simulink model "F16ASYM_Controlled_AoA"  (R2012b)
settings: Solver=ode3  SolverMode=SingleTasking  StartTime=0.0  StopTime=inf  FixedStep=T_sim  RelTol=1e-3
InitFcn:
  | load('NN_c_weights_Last_stable.mat')
values from neighbouring files (symbols this model uses):
  K_b_AoA = params(3)    [Cost_function.m]
  K_b_q = params(4)    [Cost_function.m]
  learning = 20    [Scheduling_desing.m]
  Model_used_flag = 1    [Scheduling_desing.m]
  reg_param = 0.5    [Scheduling_desing.m]
  T_sim = 0.02    [Scheduling_desing.m]
  tau_AoA = params(1)    [Cost_function.m]
  tau_q = params(2)    [Cost_function.m]
  Theta_1_roll_last = [0.00183613313267 0.00115998993235 0.0006676025148 0.00194921904952 0.00134963559861 0.00034352059664 0.000447169388141 0.00146749660935 0.00110199952389 7.77922383894e-05 0.00109492833348 0.00192687590535 ... (360 elements, 30x12)]    [NN_i_weights_LAST_STABLE.mat]
  Theta_2_roll_last = [0.000469743069697 0.000355923851088 0.00180035760697 0.00191855117771 0.00118851504447 0.0013331642065 0.0013164316578 0.000643981263341 0.00176817665434 0.000113802099363 0.000426534542462 0.00113815782354 ... (620 elements, 20x31)]    [NN_i_weights_LAST_STABLE.mat]
  Theta_3_roll_last = [9.62071520568e-05 -0.000389870886846 2.08260845013e-05 0.000140787743673 -0.000917525755397 -0.0014324207578 -0.00154701573815 -0.00131544476264 -0.00101205584381 5.06515794689e-05 -0.00111443483676 -0.00143957416141 ... (21 elements, 1x21)]    [NN_i_weights_LAST_STABLE.mat]
  V_long_lastA_w_z = [0.352826086601 -0.253633004548 -0.642535042878 0.237749930435 -0.618390629538 0.858074761295 0.268211230628 -0.448715080196 -0.0406384631192 0.401147605577 0.60598427709 0.0500551915851 ... (300 elements, 30x10)]    [NN_i_weights_LAST_STABLE.mat]
  V_long_lastAoA = [0.0774300162379 0.0911421319631 0.0352371192557 0.0542170286952 0.0651171200844 0.0177112012707 0.0982957728448 0.000259994642558 0.0194724569123 0.0466321328252 0.0556687953852 0.0252668067142 ... (300 elements, 30x10)]    [NN_i_weights_LAST_STABLE.mat]
  V_roll_last = [0.0540918675943 0.0557493347212 0.0839792276608 0.0460576391794 0.0671229058124 0.100220403067 0.0722493281881 0.0648875457457 0.00447599349201 0.0607299103823 0.0488037966361 0.0176785979393 ... (360 elements, 30x12)]    [NN_i_weights_LAST_STABLE.mat]
  V_yaw_last = [0.0965149149679 0.00833616709545 0.0365734360076 0.0523944217566 0.00790252078455 0.0700053845887 0.0345164868709 0.0111568465295 0.094060639546 0.0205483560006 0.000798047494256 0.0862769385758 ... (360 elements, 30x12)]    [NN_i_weights_LAST_STABLE.mat]
  velocity = M_eval_sche(I,J)*a    [Scheduling_desing.m]
  W_long_lastA_w_z = [-0.0522913429974 0.00385484301394 -0.00465489482472 -0.0139416219936 0.00295196421483 -0.013027768541 0.00585545058915 0.00278802233571 -0.00906272782329 -0.000396112031465 0.00405849743321 0.00509668457818 ... (31 elements, 1x31)]    [NN_i_weights_LAST_STABLE.mat]
  W_long_lastAoA = [-0.0192589013922 0.00873109909713 0.00432649597332 0.0420946902441 0.0293366820194 0.0351497798191 0.0234952374236 0.0360841187718 0.0112233388211 0.030147202199 0.0369533138617 0.00218839076415 ... (31 elements, 1x31)]    [NN_i_weights_LAST_STABLE.mat]
  W_roll_last = [-0.0006515532842 0.000535485585715 0.000550946920743 0.000806030945453 0.00045976209382 0.00065557954304 0.000945902185602 0.00070191398535 0.000635215543728 4.66501377412e-05 0.000597079583757 0.000485790566765 ... (31 elements, 1x31)]    [NN_i_weights_LAST_STABLE.mat]
  W_yaw_last = [-4.34263633305e-05 8.83823048922e-05 1.65575463724e-05 3.60293102233e-05 5.19752447623e-05 7.06399280852e-06 7.02425975821e-05 3.62680255076e-05 1.29996379937e-05 8.05072914397e-05 2.39941870661e-05 2.52427840574e-06 ... (31 elements, 1x31)]    [NN_i_weights_LAST_STABLE.mat]
undefined symbols (not defined in the file or in its folder): a1, alpha_map_eval, B, beta_map_eval, C_L_0, DiscIntNeverNeededParam, fi_flag_Simulink, G_eval, H_sq, H_sq_autotrim, k_B, m_B, M_sq, M_sq_autotrim, sigbuilder_block, Stall_curve, trim_control, trim_state, trim_throttle, V_Comp_A_w_z_last, V_Comp_last, V_roll_lastMOD, W_Comp_A_w_z_last, W_Comp_last, W_roll_lastMOD
libraries: Adaptive_FaultTolerantControl x43, dspsigops x29, F16_Actuator_Library x14, simulink x8, aerolibatmos2 x7, dsparch4 x6, simulink_extras x5, aerolibtransform2 x5, qcatlib x4, dspmtrx3 x3, dspvision x2, dspsnks4 x2
(part 4 of 11)

== system F16ASYM_Controlled_AoA/Primary Controller/P controller + adaptive Crossed NN + AWU+Lim  ==
  A_w_z des : Inport
  AoA des (rad) : Inport  Port=2
  p des (rad/s) : Inport  Port=3
  beta des (rad) : Inport  Port=4
  Anti-windup A_w_z : Inport  Port=5
  Anti-windup AoA : Inport  Port=6
  Anti-windup beta : Inport  Port=7
  All measures : Inport  Port=8
  Anti-windup signals : Inport  Port=9
  Body Rates Controller : Subsystem
  Bus Creator : BusCreator  Inputs=3
  Bus Creator1 : BusCreator  Inputs=3
  Bus Creator2 : BusCreator
  Bus Creator3 : BusCreator  Inputs=2
  Bus Selector3 : BusSelector  OutputSignals=signal1.SS meas (rad)
  Complete crossed On-line (adaptive) multi-layer NN : Subsystem  Variant=on  OverrideUsingVariant=NN on AoA
      mask Display:
      | image(imread('ANN.png'))
      | 
      | port_label('input', 1, 'v prev')
      | port_label('input', 2, 'All meas')
      | port_label('input', 3, 'NN vars')
      | port_label('input', 4, 'Anti-windup')
      | 
      | port_label('output', 1, 'v_ad^')
  Constant : Constant  Value=NaN
  Display{,1..3,5..6} (6 alike) : Display
  "Display4 " : Display
  Lat_dir Dyn Inversion: beta_dot->r_c : Subsystem
  Long Dyn Inversion: alpha_dot ->q : Subsystem
  Longitudinal Controller: AoA or A_w_z : Subsystem  Variant=on  OverrideUsingVariant=Controller of AoA
  Memory : Memory  X0=[0,0,0]
  Physical limitation : Subsystem
  Ref Model and P Controller : Adaptive_FaultTolerantControl/Ref Model and P Controller  tau=0.45  y_i=trim_state(9)  K_f=1  K_b=5
  Scope1 : Scope
      settings: YMin=-8000  YMax=9000  SaveName=ScopeData27
  "Sigmoid " : Subsystem  mask{a=0.15}
      mask prompts: a "Sigmoid a param"
      mask TypeOptions a: a/Value
      mask Display:
      | x=-25:0.1:25;
      | 
      | y=(2.0 ./ (1.0 + exp(-a.*x))-1) ;
      | y2=zeros(size(x));
      | 
      | plot(x,y,x,y2);
      | 
      | text(-12,0.5, ['a= ',num2str(a)])
  Sum : Sum  Inputs=-+|
  Sum1 : Sum  Inputs=+-|
  Terminator1 : Terminator
  Angular acc des : Outport
  Control_in : Outport  Port=2
  wires:
  Lat_dir Dyn Inversion: beta_dot->r_c/1(r_c) -> Display6/1, Body Rates Controller/3(r_ref)
  Bus Selector3/1 -> Ref Model and P Controller/2  "<SS meas (rad)>"
  p des (rad/s)/1 -> Body Rates Controller/1(p_ref)
  Long Dyn Inversion: alpha_dot ->q/1(q_c) -> Body Rates Controller/2(q_ref), Display1/1
  beta des (rad)/1 -> Ref Model and P Controller/1
  Longitudinal Controller: AoA or A_w_z/3(alpha_dot_c) -> Long Dyn Inversion: alpha_dot ->q/1(alpha_dot_c), Display/1
  AoA des (rad)/1 -> Longitudinal Controller: AoA or A_w_z/2(AoA des (rad))
  Anti-windup AoA/1 -> Longitudinal Controller: AoA or A_w_z/4(Anti-windup AoA)
  Anti-windup A_w_z/1 -> Longitudinal Controller: AoA or A_w_z/3(Anti-windup A_w_z)
  A_w_z des/1 -> Longitudinal Controller: AoA or A_w_z/1(A_w_z des)
  Sum/1 -> "Display4 "/1, "Sigmoid "/1(In), Physical limitation/1(v comm)  "v"
  All measures/1 -> Complete crossed On-line (adaptive) multi-layer NN/2(All_meas), Physical limitation/2(all meas), Body Rates Controller/4(All_meas), Lat_dir Dyn Inversion: beta_dot->r_c/2(All_meas), Bus Selector3/1, Long Dyn Inversion: alpha_dot ->q/2(All_meas), Longitudinal Controller: AoA or A_w_z/5(All meas)
  Body Rates Controller/4(Angular acc des (rad/s^2)) -> Display3/1, Sum/2  "v_p+v_dot_ff"
  Bus Creator/1 -> Complete crossed On-line (adaptive) multi-layer NN/3(NN variables)
  Memory/1 -> Complete crossed On-line (adaptive) multi-layer NN/1(v_ad^ prev)
  Body Rates Controller/2(p_chanel vars) -> Bus Creator/2  "p_chanel_vars"
  Body Rates Controller/1(q_chanel vars) -> Bus Creator1/3  "q_chanel_vars"
  Longitudinal Controller: AoA or A_w_z/1(A_chanel vars) -> Bus Creator1/1  "A_chanel vars"
  Longitudinal Controller: AoA or A_w_z/2(alpha_chanel vars) -> Bus Creator1/2  "alpha_chanel vars"
  Bus Creator1/1 -> Bus Creator/1  "Long chanel"
  Ref Model and P Controller/2 -> Bus Creator2/1  "beta_sf_dot"
  Ref Model and P Controller/3 -> Sum1/1, Bus Creator2/2  "beta_sf"
  Sum1/1 -> Bus Creator2/3  "beta_err"
  Ref Model and P Controller/4 -> Sum1/2
  Ref Model and P Controller/5 -> Bus Creator2/4  "K_b_beta"
  Body Rates Controller/3(r_chanel vars) -> Bus Creator3/1  "r_chanel vars"
  Bus Creator2/1 -> Bus Creator3/2  "beta_chanel vars"
  Bus Creator3/1 -> Bus Creator/3  "beta_r_chanel"
  Anti-windup beta/1 -> Terminator1/1
  "Sigmoid "/1(Out) -> Memory/1
  Complete crossed On-line (adaptive) multi-layer NN/1(v_ad^) -> Scope1/1, Display2/1, Sum/1  "v_ad^"
  Ref Model and P Controller/1 -> Display5/1, Lat_dir Dyn Inversion: beta_dot->r_c/1(beta_dot_c)
  Anti-windup signals/1 -> Complete crossed On-line (adaptive) multi-layer NN/4(AWU)
  Physical limitation/1(v limted) -> Angular acc des/1
  Constant/1 -> Control_in/1

== system F16ASYM_Controlled_AoA/Primary Controller/P controller + adaptive Isolated NN ==
  A_w_z des : Inport
  AoA des (rad) : Inport  Port=2
  p des (rad/s) : Inport  Port=3
  beta des (rad) : Inport  Port=4
  Anti-windup A_w_z : Inport  Port=5
  Anti-windup AoA : Inport  Port=6
  Anti-windup beta : Inport  Port=7
  All measures : Inport  Port=8
  Anti-windup signals : Inport  Port=9
  Body Rates Controller : Subsystem
  Bus Creator : BusCreator  Inputs=3
  Bus Creator1 : BusCreator  Inputs=3
  Bus Creator2 : BusCreator
  Bus Creator3 : BusCreator  Inputs=2
  Bus Selector3 : BusSelector  OutputSignals=signal1.SS meas (rad)
  Display{,1..6} (7 alike) : Display
  Ground : Ground
  Lat_dir Dyn Inversion: beta_dot->r_c : Subsystem
  Long Dyn Inversion: alpha_dot ->q : Subsystem
  Longitudinal Controller: AoA or A_w_z : Subsystem  Variant=on  OverrideUsingVariant=Controller of A_w_z
  Memory : Memory  X0=[0,0,0]
  On-line (adaptive) multi-layer NNs : Subsystem
      mask Display:
      | image(imread('ANN.png'))
      | 
      | port_label('input', 1, 'v prev')
      | port_label('input', 2, 'All meas')
      | port_label('input', 3, 'NN vars')
      | 
      | port_label('output', 1, 'v_ad^')
  On-line (adaptive) multi-layer NNs SIMPL : Subsystem  Commented=on
      mask Display:
      | image(imread('ANN.png'))
      | 
      | port_label('input', 1, 'v prev')
      | port_label('input', 2, 'All meas')
      | port_label('input', 3, 'NN vars')
      | 
      | port_label('output', 1, 'v_ad^')
  Ref Model and P Controller : Adaptive_FaultTolerantControl/Ref Model and P Controller  tau=0.45  y_i=trim_state(9)  K_f=1  K_b=5
  "Sigmoid " : Subsystem  mask{a=0.15}
      mask prompts: a "Sigmoid a param"
      mask TypeOptions a: a/Value
      mask Display:
      | x=-25:0.1:25;
      | 
      | y=(2.0 ./ (1.0 + exp(-a.*x))-1) ;
      | y2=zeros(size(x));
      | 
      | plot(x,y,x,y2);
      | 
      | text(-12,0.5, ['a= ',num2str(a)])
  Sum : Sum  Inputs=-+|
  Sum1 : Sum  Inputs=+-|
  Terminator : Terminator
  Terminator1 : Terminator
  Angular acc des : Outport
  Control_in : Outport  Port=2
  wires:
  Lat_dir Dyn Inversion: beta_dot->r_c/1(r_c) -> Display6/1, Body Rates Controller/3(r_ref)
  Bus Selector3/1 -> Ref Model and P Controller/2  "<SS meas (rad)>"
  p des (rad/s)/1 -> Body Rates Controller/1(p_ref)
  Long Dyn Inversion: alpha_dot ->q/1(q_c) -> Display1/1, Body Rates Controller/2(q_ref)
  beta des (rad)/1 -> Ref Model and P Controller/1
  Longitudinal Controller: AoA or A_w_z/3(alpha_dot_c) -> Long Dyn Inversion: alpha_dot ->q/1(alpha_dot_c), Display/1
  AoA des (rad)/1 -> Longitudinal Controller: AoA or A_w_z/2(AoA des (rad))
  Anti-windup AoA/1 -> Longitudinal Controller: AoA or A_w_z/4(Anti-windup AoA)
  Anti-windup A_w_z/1 -> Longitudinal Controller: AoA or A_w_z/3(Anti-windup A_w_z)
  A_w_z des/1 -> Longitudinal Controller: AoA or A_w_z/1(A_w_z des)
  Sum/1 -> Display4/1, "Sigmoid "/1(In), Angular acc des/1  "v"
  Body Rates Controller/4(Angular acc des (rad/s^2)) -> Display3/1, Sum/2  "v_p+v_dot_ff"
  Bus Creator/1 -> On-line (adaptive) multi-layer NNs/3(NN variables)
  Memory/1 -> On-line (adaptive) multi-layer NNs/1(v_ad^ prev)
  Body Rates Controller/2(p_chanel vars) -> Bus Creator/2  "p_chanel_vars"
  Body Rates Controller/1(q_chanel vars) -> Bus Creator1/3  "q_chanel_vars"
  Longitudinal Controller: AoA or A_w_z/1(A_chanel vars) -> Bus Creator1/1  "A_chanel vars"
  Longitudinal Controller: AoA or A_w_z/2(alpha_chanel vars) -> Bus Creator1/2  "alpha_chanel vars"
  Bus Creator1/1 -> Bus Creator/1  "Long chanel"
  Ref Model and P Controller/2 -> Bus Creator2/1  "beta_sf_dot"
  Ref Model and P Controller/3 -> Sum1/1, Bus Creator2/2  "beta_sf"
  Sum1/1 -> Bus Creator2/3  "beta_err"
  Ref Model and P Controller/4 -> Sum1/2
  Ref Model and P Controller/5 -> Bus Creator2/4  "K_b_beta"
  Body Rates Controller/3(r_chanel vars) -> Bus Creator3/1  "r_chanel vars"
  Bus Creator2/1 -> Bus Creator3/2  "beta_chanel vars"
  Bus Creator3/1 -> Bus Creator/3  "beta_r_chanel"
  Anti-windup beta/1 -> Terminator1/1
  "Sigmoid "/1(Out) -> Memory/1
  On-line (adaptive) multi-layer NNs/1(v_ad^) -> Sum/1, Display2/1  "v_ad^"
  Ref Model and P Controller/1 -> Display5/1, Lat_dir Dyn Inversion: beta_dot->r_c/1(beta_dot_c)
  All measures/1 -> On-line (adaptive) multi-layer NNs/2(All_meas), Body Rates Controller/4(All_meas), Lat_dir Dyn Inversion: beta_dot->r_c/2(All_meas), Bus Selector3/1, Long Dyn Inversion: alpha_dot ->q/2(All_meas), Longitudinal Controller: AoA or A_w_z/5(All meas)
  Anti-windup signals/1 -> Terminator/1
  Ground/1 -> Control_in/1

== system F16ASYM_Controlled_AoA/Primary Controller/PI Primary Controller ==
  A_w_z des : Inport
  AoA des (rad) : Inport  Port=2
  p des (rad/s) : Inport  Port=3
  beta des (rad) : Inport  Port=4
  Anti-windup A_w_z : Inport  Port=5
  Anti-windup AoA : Inport  Port=6
  Anti-windup beta : Inport  Port=7
  All measures : Inport  Port=8
  Anti-windup signals : Inport  Port=9
  Body Rates Controller : Subsystem
  Bus Selector3 : BusSelector  OutputSignals=signal1.SS meas (rad)
  Display{,1..3} (4 alike) : Display
  Ground : Ground
  Lat_dir Dyn Inversion: beta_dot->r_c : Subsystem
  Long Dyn Inversion: alpha_dot ->q : Subsystem
  Longitudinal Controller: AoA or A_w_z : Subsystem  Variant=on  OverrideUsingVariant=Controller of A_w_z
  PI Controller: beta  controller : Adaptive_FaultTolerantControl/PI Controller  delta=0  K_a=0  y_i=trim_state(9)  Des_way=auto  omega_n=2  xi=1  Z1=-50  K_b=6  f_i=0.25  f_c=1
  Angular acc des : Outport
  Control_in : Outport  Port=2
  wires:
  A_w_z des/1 -> Longitudinal Controller: AoA or A_w_z/1(A_w_z des)
  Anti-windup A_w_z/1 -> Longitudinal Controller: AoA or A_w_z/3(Anti-windup A_w_z)
  Anti-windup AoA/1 -> Longitudinal Controller: AoA or A_w_z/4(Anti-windup AoA)
  AoA des (rad)/1 -> Longitudinal Controller: AoA or A_w_z/2(AoA des (rad))
  Longitudinal Controller: AoA or A_w_z/1(alpha_dot_c) -> Display/1, Long Dyn Inversion: alpha_dot ->q/1(alpha_dot_c)
  All measures/1 -> Bus Selector3/1, Lat_dir Dyn Inversion: beta_dot->r_c/2(All_meas), Body Rates Controller/4(All_meas), Longitudinal Controller: AoA or A_w_z/5(All meas), Long Dyn Inversion: alpha_dot ->q/2(All_meas)
  Anti-windup beta/1 -> PI Controller: beta  controller/3
  beta des (rad)/1 -> PI Controller: beta  controller/1
  Long Dyn Inversion: alpha_dot ->q/1(q_c) -> Body Rates Controller/2(q_ref), Display1/1
  p des (rad/s)/1 -> Body Rates Controller/1(p_ref)
  Body Rates Controller/1(Angular acc des (rad/s^2)) -> Angular acc des/1
  PI Controller: beta  controller/1 -> Lat_dir Dyn Inversion: beta_dot->r_c/1(beta_dot_c), Display3/1
  Anti-windup signals/1 -> Body Rates Controller/5(All Anti-windup signals)
  Bus Selector3/1 -> PI Controller: beta  controller/2  "<SS meas (rad)>"
  Lat_dir Dyn Inversion: beta_dot->r_c/1(r_c) -> Body Rates Controller/3(r_ref), Display2/1
  Ground/1 -> Control_in/1

== system F16ASYM_Controlled_AoA/SI and FDI/SI and FDI: Realistic ==
  note: RECONFIGURATION PARAMETERS
      |
      | 24. mass  Estimated mass
      | 25. S_current_L
      | 26. S_current_R
      | 27. S_fin_current
      | 28. x_cg
      | 29. Jy
      | 30. Jxz
      | 31. Jz
      | 32. Jx
      | 33. EFF_el_L
      | 34. EFF_el_R
      | 35. EFF_ail_L
      | 36. EFF_ail_R
      | 37. EFF_rud
      | 38. EFF_lef_L
      | 39. EFF_lef_R
      | 40. Delta_C_Lift_X
      | 41. Delta_C_Drag_X
      | 42. Delta_C_m_X
  Inexistent Reconfig bus : Inport
  Control comms : Inport  Port=2
  All  meas : Inport  Port=3
  Bus Creator : BusCreator  Inputs=3
  FDI: Assumed? : Subsystem  VariantObject=FDI: Realsitic
  Mass props : Selector  InputPortWidth=6  IndexOptions=Index vector (dialog)  Indices=2:6  OutputSizes=1
  Mux : Mux  Inputs=[9 7 3]
  Mux1 : Mux  Inputs=3
  SI : Subsystem
  mass : Selector  InputPortWidth=6  IndexOptions=Index vector (dialog)  Indices=1  OutputSizes=1
  Est reconf params : Outport
  wires:
  All  meas/1 -> FDI: Assumed?/2(All  meas), SI/2(All meas)
  FDI: Assumed?/3(Effectiveness) -> SI/1(Control Eff), Mux/2
  Mux/1 -> Bus Creator/3  "Reconfig signal"
  FDI: Assumed?/2(Blockades now) -> Bus Creator/2
  FDI: Assumed?/1(Blockades at) -> Bus Creator/1
  Bus Creator/1 -> Est reconf params/1
  Inexistent Reconfig bus/1 -> FDI: Assumed?/1(Inexistent Reconfig bus)
  Control comms/1 -> SI/3(Control comms)
  mass/1 -> Mux1/1
  SI/2(Est Surfs) -> Mux1/2
  Mass props/1 -> Mux1/3
  SI/1(Est Mass props) -> Mass props/1, mass/1
  Mux1/1 -> Mux/1
  SI/3(Est Aero changes) -> Mux/3

== system F16ASYM_Controlled_AoA/SI and FDI/SI and FDI: Unrealistic ==
  Inexistent Reconfig bus : Inport
  Control comms : Inport  Port=2
  All  meas : Inport  Port=3
  Terminator : Terminator
  Terminator1 : Terminator
  Est reconf params : Outport
  wires:
  Inexistent Reconfig bus/1 -> Est reconf params/1
  All  meas/1 -> Terminator/1
  Control comms/1 -> Terminator1/1

== system F16ASYM_Controlled_AoA/Speed-Throttle control/Stall protection TAS ==
  note: Margin here?
  TAS comm : Inport
  All meas : Inport  Port=2
  Bus Selector : BusSelector  OutputSignals=signal1.Alt meas (m),signal2.a
  Display : Display
  Gain2 : Gain  Gain=1.2
  Min TAS : Product  Inputs=**
  MinMax : MinMax  Function=max  Inputs=2
  Stall curve 1g : Lookup_n-D  NumberOfTableDimensions=1  BreakpointsForDimension1=Stall_curve.H_2  Table=Stall_curve.M_2  RemoveProtectionInput=on  RndMeth=Simplest  InputSameDT=on
  TAS des : Outport
  tag scope: Min_Mach=global
  wires:
  MinMax/1 -> TAS des/1
  TAS comm/1 -> MinMax/2
  All meas/1 -> Bus Selector/1
  Bus Selector/1 -> Stall curve 1g/1  "<Alt meas (m)>"
  Stall curve 1g/1 -> [Min_Mach], Min TAS/1  "Min M"
  Bus Selector/2 -> Min TAS/2  "<a>"
  Min TAS/1 -> Gain2/1
  Gain2/1 -> Display/1, MinMax/1

== system F16ASYM_Controlled_AoA/Speed-Throttle control/Throttle controller ==
  V_TAS des : Inport
  All meas : Inport  Port=2
  Add : Sum  Inputs=|+-
  Bus Selector : BusSelector  OutputSignals=signal1.V_TAS (m/s)
  Mux : Mux  Inputs=2
  PID Controller2 : simulink/Continuous/PID Controller  Controller=P  TimeDomain=Continuous-time  SampleTime=1  IntegratorMethod=Forward Euler  FilterMethod=Forward Euler  Form=Parallel  P=0.8  I=0.0001  D=-0.01  N=100  InitialConditionSource=internal  InitialConditionForIntegrator=0  InitialConditionForFilter=0  ExternalReset=none  LimitOutput=on  UpperSaturationLimit=1  LowerSaturationLimit=0  LinearizeAsGain=on  AntiWindupMode=back-calculation  Kb=3  TrackingMode=off  Kt=1  PParamMin=[]  PParamMax=[]  IParamMin=[]  IParamMax=[]  DParamMin=[]  DParamMax=[]  NParamMin=[]  NParamMax=[]  KbParamMin=[]  KbParamMax=[]  KtParamMin=[]  KtParamMax=[]  POutMin=[]  POutMax=[]  IOutMin=[]  IOutMax=[]  DOutMin=[]  DOutMax=[]  NOutMin=[]  NOutMax=[]  KbOutMin=[]  KbOutMax=[]  KtOutMin=[]  KtOutMax=[]  IntegratorOutMin=[]  IntegratorOutMax=[]  FilterOutMin=[]  FilterOutMax=[]  SumOutMin=[]  SumOutMax=[]  SumI1OutMin=[]  SumI1OutMax=[]  SumI2OutMin=[]  SumI2OutMax=[]  SumI3OutMin=[]  SumI3OutMax=[]  SumDOutMin=[]  SumDOutMax=[]  SaturationOutMin=[]  SaturationOutMax=[]  IntegratorContinuousStateAttributes=''  IntegratorStateMustResolveToSignalObject=off  IntegratorRTWStateStorageClass=Auto  FilterContinuousStateAttributes=''  FilterStateMustResolveToSignalObject=off  FilterRTWStateStorageClass=Auto
  Scope : Scope
      settings: YMin=152.5  YMax=207.5  SaveName=ScopeData30
  Scope1 : Scope
      settings: YMin=1  YMax=1  SaveName=ScopeData31
  Throttle des : Outport
  wires:
  All meas/1 -> Bus Selector/1
  V_TAS des/1 -> Mux/1, Add/1
  Bus Selector/1 -> Mux/2, Add/2  "<V_TAS (m/s)>"
  PID Controller2/1 -> Scope1/1, Throttle des/1
  Add/1 -> PID Controller2/1
  Mux/1 -> Scope/1

== system F16ASYM_Controlled_AoA/Stall protection A_z and AoA/AoA and load factor map ==
  Reconf param : Inport
  All meas : Inport  Port=2
  A_w_z comm : Inport  Port=3
  AoA comm : Inport  Port=4
  2-D Lookup Table : Lookup_n-D  BreakpointsForDimension1=M_sq  BreakpointsForDimension2=H_sq  Table=G_eval  RemoveProtectionInput=on  SampleTime=5*T_sim  RndMeth=Simplest  InputSameDT=on
  Bias : Bias  Bias=1
  Bus Selector : BusSelector  OutputSignals=signal2.Mach,signal1.Alt meas (m),signal1.AoA meas (rad),signal2.A_w_CG
  Constant : Constant  Value=0
  Display : Display
  Display1 : Display
  Gain : Gain  Gain=-1
  Gain1 : Gain  Gain=-1
  Gain2 : Gain  Gain=9.81
  If : If  NumInputs=4  IfExpression=u1>=17 | (u1<=-17) | (u2>=u3) | (u2<=u4)  SampleTime=T_sim
  If Action Subsystem : Subsystem  TreatAsAtomicUnit=on
  Radians to Degrees : simulink_extras/Transformations/Radians to Degrees
  Rate Limiter : RateLimiter  RisingSlewLimit=2*9.8  FallingSlewLimit=-2*9.8  SampleTimeMode=inherited
  Rate Limiter2 : RateLimiter  RisingSlewLimit=deg2rad(15)  FallingSlewLimit=-deg2rad(15)  SampleTimeMode=inherited  InitialCondition=trim_state(8)
  Saturation : Saturate  UpperLimit=deg2rad(20)  LowerLimit=-deg2rad(20)
  Saturation Dynamic : simulink/Discontinuities/Saturation Dynamic  OutMin=[]  OutMax=[]  OutDataTypeStr=Inherit: Same as second input  OutDataType=fixdt(1, 16)  OutScaling=2^-10  DoSatur=off
  Saturation1 : Saturate  UpperLimit=10  LowerLimit=0
  Selector : Selector  InputPortWidth=3  IndexOptions=Index vector (dialog)  Indices=3  OutputSizes=1
  Switch : Switch  Threshold=0.5
  isNaN1 : RelationalOperator  Operator=isNaN  OutDataTypeStr=boolean
  A_w_z des : Outport
  AoA des : Outport  Port=2
  wires:
  If/1 -> If Action Subsystem/Action
  Switch/1 -> Gain/1, Saturation Dynamic/1, If/3, Display/1
  Constant/1 -> Switch/1
  isNaN1/1 -> Switch/2
  Gain2/1 -> isNaN1/1, Switch/3
  Saturation1/1 -> Gain2/1
  Gain1/1 -> Display1/1, If/2
  Selector/1 -> Gain1/1
  Bus Selector/4 -> Selector/1  "<A_w_CG>"
  Radians to Degrees/1 -> If/1
  Bus Selector/3 -> Radians to Degrees/1  "<AoA meas (rad)>"
  Gain/1 -> Saturation Dynamic/3, If/4
  Bias/1 -> Saturation1/1
  Saturation Dynamic/1 -> A_w_z des/1
  Rate Limiter/1 -> Saturation Dynamic/2
  Rate Limiter2/1 -> AoA des/1
  AoA comm/1 -> Saturation/1
  Bus Selector/1 -> 2-D Lookup Table/1  "<Mach>"
  2-D Lookup Table/1 -> Bias/1
  Bus Selector/2 -> 2-D Lookup Table/2  "<Alt meas (m)>"
  A_w_z comm/1 -> Rate Limiter/1
  Saturation/1 -> Rate Limiter2/1
  All meas/1 -> Bus Selector/1

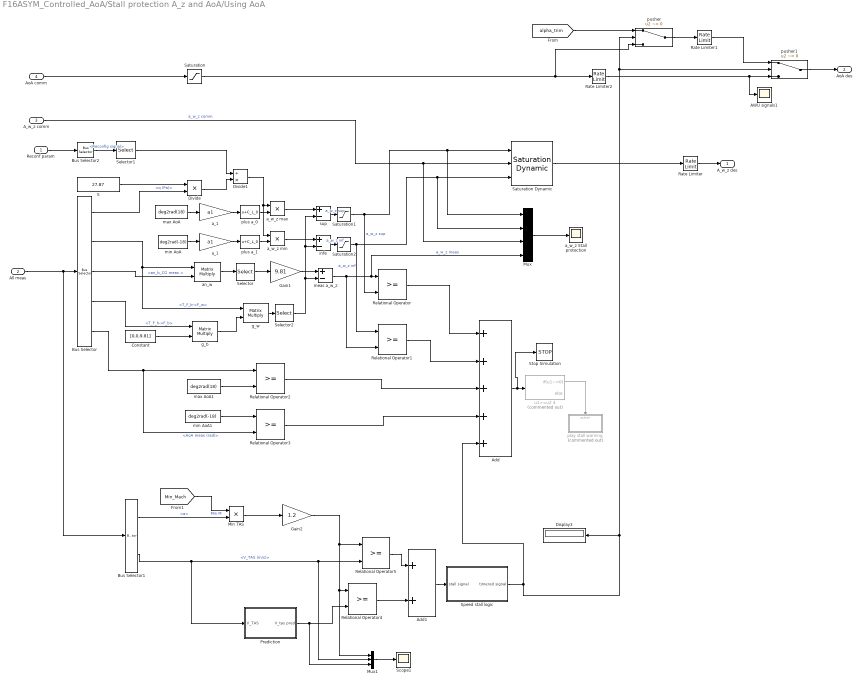
== system F16ASYM_Controlled_AoA/Stall protection A_z and AoA/Using AoA ==
  Reconf param : Inport
  All meas : Inport  Port=2
  A_w_z comm : Inport  Port=3
  AoA comm : Inport  Port=4
  AWU signals1 : Scope
      settings: TimeRange=4.5  YMin=0.005  YMax=0.05  SaveName=ScopeData39
  Add : Sum  Inputs=+++++
  Add1 : Sum
  Bus Selector : BusSelector  OutputSignals=signal2.q (Pa),signal2.T_F_b->F_w,signal1.an_b_CG meas ,signal2.T_F_h->F_b,signal1.AoA meas (rad)
  Bus Selector1 : BusSelector  OutputSignals=signal2.a,signal1.V_TAS (m/s)
  Bus Selector2 : BusSelector  OutputSignals=Reconfig signal
  Constant : Constant  Value=[0,0,9.81]
  Display3 : Display
  Divide : Product  Inputs=**
  Divide1 : Product  Inputs=/*
  Gain1 : Gain  Gain=9.81
  Gain2 : Gain  Gain=1.2
  Min TAS : Product  Inputs=**
  Mux : Mux
  Mux1 : Mux  Inputs=3
  Prediction : Subsystem  mask{T_pred=5}
      mask prompts: T_pred "Prediction time"
      mask TypeOptions T_pred: T_pred/Gain
  Rate Limiter : RateLimiter  RisingSlewLimit=4*9.8  FallingSlewLimit=-4*9.8  SampleTimeMode=inherited
  Rate Limiter1 : RateLimiter  RisingSlewLimit=deg2rad(2)  FallingSlewLimit=-deg2rad(2)  SampleTimeMode=inherited  InitialCondition=trim_state(8)
  Rate Limiter2 : RateLimiter  RisingSlewLimit=deg2rad(10)  FallingSlewLimit=-deg2rad(10)  SampleTimeMode=inherited  InitialCondition=trim_state(8)
  Relational Operator{,1..5} (6 alike) : RelationalOperator  OutDataTypeStr=boolean
  S : Constant  Value=27.87
  Saturation : Saturate  UpperLimit=deg2rad(19)  LowerLimit=-deg2rad(19)
  Saturation Dynamic : simulink/Discontinuities/Saturation Dynamic  OutMin=[]  OutMax=[]  OutDataTypeStr=Inherit: Same as second input  OutDataType=fixdt(1, 16)  OutScaling=2^-10  DoSatur=off
  Saturation1 : Saturate  UpperLimit=9*9.81  LowerLimit=0
  Saturation2 : Saturate  UpperLimit=0  LowerLimit=-5*9.81
  Scope1 : Scope
      settings: YMin=80  YMax=210  SaveName=ScopeData25
  Selector : Selector  InputPortWidth=3  IndexOptions=Index vector (dialog)  Indices=3  OutputSizes=1
  Selector1 : Selector  InputPortWidth=19  IndexOptions=Index vector (dialog)  Indices=1  OutputSizes=1
  Selector2 : Selector  InputPortWidth=3  IndexOptions=Index vector (dialog)  Indices=3  OutputSizes=1
  Speed stall logic : Subsystem
  Stop Simulation : Stop
  a_1 : Gain  Gain=a1
  "a_1  " : Gain  Gain=a1
  a_w_z Stall protection : Scope
      settings: ShowLegends=on  YMin=-225  YMax=225  SaveName=ScopeData28
  a_w_z max : Product  Inputs=**
  a_w_z min : Product  Inputs=**
  an_w : Product  Multiplication=Matrix(*)
  g_b : Product  Multiplication=Matrix(*)
  g_w : Product  Multiplication=Matrix(*)
  infe : Sum  Inputs=+-
  max AoA : Constant  Value=deg2rad(18)
  max AoA1 : Constant  Value=deg2rad(18)
  meas a_w_z : Sum  Inputs=+-
  min AoA : Constant  Value=deg2rad(-18)
  min AoA1 : Constant  Value=deg2rad(-18)
  play stall warning : Subsystem  Commented=on  TreatAsAtomicUnit=on
  plus a_0 : Bias  Bias=C_L_0
  plus a_1 : Bias  Bias=C_L_0
  pusher : Switch  Criteria=u2 ~= 0  Threshold=0.5
  pusher1 : Switch  Criteria=u2 ~= 0  Threshold=0.5
  sup : Sum  Inputs=+-
  u1>=u2 4 : If  Commented=on  IfExpression=u1~=0  SampleTime=T_sim
  A_w_z des : Outport
  AoA des : Outport  Port=2
  wires:
  AoA comm/1 -> Saturation/1
  pusher1/1 -> AoA des/1
  A_w_z comm/1 -> Mux/3, Saturation Dynamic/2  "a_w_z comm"
  All meas/1 -> Bus Selector1/1, Bus Selector/1
  [Min_Mach] -> Min TAS/1  "Min M"
  Bus Selector1/1 -> Min TAS/2  "<a>"
  Reconf param/1 -> Bus Selector2/1
  S/1 -> Divide/1
  Bus Selector/1 -> Divide/2  "<q (Pa)>"
  Bus Selector2/1 -> Selector1/1  "<Reconfig signal>"
  Selector1/1 -> Divide1/1
  Divide/1 -> Divide1/2
  a_1/1 -> plus a_0/1
  Divide1/1 -> a_w_z min/1, a_w_z max/1
  plus a_0/1 -> a_w_z max/2
  Bus Selector/3 -> an_w/2  "<an_b_CG meas >"
  Bus Selector/2 -> g_w/1, an_w/1  "<T_F_b->F_w>"
  Selector/1 -> Gain1/1
  an_w/1 -> Selector/1
  Bus Selector/4 -> g_b/1  "<T_F_h->F_b>"
  Constant/1 -> g_b/2
  g_b/1 -> g_w/2
  a_w_z max/1 -> sup/1
  g_w/1 -> Selector2/1
  Gain1/1 -> meas a_w_z/1
  Rate Limiter/1 -> A_w_z des/1
  a_w_z min/1 -> infe/1
  Selector2/1 -> meas a_w_z/2, infe/2, sup/2
  "a_1  "/1 -> plus a_1/1
  plus a_1/1 -> a_w_z min/2
  max AoA/1 -> a_1/1
  min AoA/1 -> "a_1  "/1
  sup/1 -> Saturation1/1  "a_w_z sup"
  infe/1 -> Saturation2/1  "a_w_z inf"
  Bus Selector/5 -> Relational Operator3/2, Relational Operator2/1  "<AoA meas (rad)>"
  max AoA1/1 -> Relational Operator2/2
  min AoA1/1 -> Relational Operator3/1
  Mux/1 -> a_w_z Stall protection/1
  Bus Selector1/2 -> Mux1/2, Relational Operator5/2, Prediction/1(V_TAS)  "<V_TAS (m/s)>"
  Gain2/1 -> Mux1/1, Relational Operator4/1, Relational Operator5/1
  Relational Operator/1 -> Add/1
  Relational Operator1/1 -> Add/2
  Relational Operator2/1 -> Add/3
  Relational Operator3/1 -> Add/4
  meas a_w_z/1 -> Relational Operator1/2, Mux/4, Relational Operator/1  "a_w_z meas"
  Add/1 -> Stop Simulation/1, u1>=u2 4/1
  Saturation/1 -> pusher/3, Rate Limiter2/1
  [alpha_trim] -> pusher/1
  Saturation Dynamic/1 -> Rate Limiter/1
  Saturation1/1 -> Relational Operator/2, Mux/1, Saturation Dynamic/1  "a_w_z sup"
  Saturation2/1 -> Relational Operator1/1, Mux/2, Saturation Dynamic/3  "a_w_z inf"
  Min TAS/1 -> Gain2/1
  Prediction/1(V_tas pred) -> Mux1/3, Relational Operator4/2
  Relational Operator5/1 -> Add1/1
  Relational Operator4/1 -> Add1/2
  Add1/1 -> Speed stall logic/1(stall signal)
  Mux1/1 -> Scope1/1
  pusher/1 -> Rate Limiter1/1
  Rate Limiter2/1 -> AWU signals1/1, pusher1/3
  Rate Limiter1/1 -> pusher1/1
  Speed stall logic/1(timered signal) -> Display3/1, pusher/2, pusher1/2, Add/5
  u1>=u2 4/1 -> play stall warning/Action

== system F16ASYM_Controlled_AoA/Anti-windup Calculation/Anti-windup: NO reconfigurable/Moments ==
  C_L : Inport
  C_M : Inport  Port=2
  C_N : Inport  Port=3
  q : Inport  Port=4
  B span : Constant  Value=9.144
  CMA : Constant  Value=3.45
  Divide : Product  Inputs=**
  Divide1 : Product  Inputs=***
  Divide2 : Product  Inputs=**
  Divide3 : Product  Inputs=***
  Divide4 : Product  Inputs=**
  S_w : Constant  Value=27.87
  S_w1 : Constant  Value=27.87
  q1 : InportShadow  Port=4
  L : Outport
  M : Outport  Port=2
  N : Outport  Port=3
  wires:
  Divide4/1 -> M/1  "M"
  Divide3/1 -> Divide4/2
  C_M/1 -> Divide4/1
  CMA/1 -> Divide3/3
  S_w1/1 -> Divide3/2
  q1/1 -> Divide3/1
  Divide2/1 -> N/1  "N"
  C_N/1 -> Divide2/2
  Divide/1 -> L/1  "L"
  Divide1/1 -> Divide/2, Divide2/1
  C_L/1 -> Divide/1
  B span/1 -> Divide1/3
  S_w/1 -> Divide1/2
  q/1 -> Divide1/1

== matlab function F16ASYM_Controlled_AoA/Primary Controller/P  + Crossed NN + AWU+Lim + hand-over/P controller + adaptive Crossed NN + AWU+Lim   in AoA/Complete crossed On-line (adaptive) multi-layer NN: AoA/Cross NN ==
  data: X_bar input size=[25,1]; v_ad_comp output; e input; K_roll input; Ks_long input; Ks_yaw input; B input; Learnign_rate input size=1; Reg_param input size=1; AWU input; W input size=[3,51]; V input size=[50,25]; v_ad output; Z_norm_unit output; T_sim parameter; W_update output; V_update output
function [v_ad_comp,v_ad,Z_norm_unit,W_update,V_update]  = Cross_NN(X_bar,e, K_roll,Ks_long,Ks_yaw,B,Learnign_rate,Reg_param,AWU,W,V,T_sim)

%% Compute prelimiary parametes
P_roll=1/K_roll;
P_long = [   1/Ks_long(1) , 1/(Ks_long(1)^2+Ks_long(1)*Ks_long(2));
     1/(Ks_long(1)^2+Ks_long(1)*Ks_long(2)) ,(Ks_long(1)^2+Ks_long(1)*Ks_long(2)+1)/(Ks_long(2)^2*Ks_long(1)+Ks_long(2)*Ks_long(1)^2) ];
P_yaw = [   1/Ks_yaw(1) , 1/(Ks_yaw(1)^2+Ks_yaw(1)*Ks_yaw(2));
     1/(Ks_yaw(1)^2+Ks_yaw(1)*Ks_yaw(2)) ,(Ks_yaw(1)^2+Ks_yaw(1)*Ks_yaw(2)+1)/(Ks_yaw(2)^2*Ks_yaw(1)+Ks_yaw(2)*Ks_yaw(1)^2) ];
 
 P = blkdiag(P_roll,P_long,P_yaw);



zeta= e'*P*B;
% Introduce Anti-windup
K_awu = 1.2;
zeta = zeta - K_awu*AWU'.*T_sim; 
% if norm(AWU)~=0
%     Learnign_rate=0;
% end
% Convergence limitation
if norm(zeta)>2/(T_sim*Learnign_rate*Reg_param)
    zeta = (zeta./norm(zeta)).*(1.8/(T_sim*Learnign_rate*Reg_param));
end
%% Feedforward
z = V*X_bar;
s=sigmoid(V*X_bar);

sigma = [1 ; s ];
% v_ad = W*sigma;

sigma_grad = (sigma.*(ones(size(sigma))-sigma));

%% Compute the gradients or adaptation laws
Gamma_w= Learnign_rate; % W learnign rate
Gamma_v= Learnign_rate; %V learning rate
lambda = Reg_param;

V_dot=zeros(size(V));
W_dot=zeros(size(W));

W_dot= -Gamma_w*(  (sigma - sigma_grad.*[1;z] )*zeta  )';
W_dot(:,2:end)= W_dot(:,2:end) - Gamma_w*lambda*norm(zeta)*(W(:,2:end));

M = W'*zeta'.*sigma_grad ;
V_dot= -Gamma_v*( M(2:end)*X_bar'  );
V_dot(:,2:end)= V_dot(:,2:end) - Gamma_v*lambda*norm(zeta).*V(:,2:end);


% % % % Other way: Based on notes of Andrew NG
% % % 
% % % delta2=W'*zeta'.*sigma_grad;
% % % 
% % % V_dot = - Gamma_v*( delta2(2:end)*X_bar');
% % % V_dot(:,2:end)= V_dot(:,2:end) - Gamma_v*lambda*norm(zeta).*V(:,2:end);
% % % 
% % % W_dot = - Gamma_w*( sigma*zeta)';
% % % W_dot(:,2:end)= W_dot(:,2:end) - Gamma_w*lambda*norm(zeta)*(W(:,2:end));



%% Adaptation
W_update = W + T_sim*W_dot;
V_update = V + T_sim*V_dot;

%% Re-compute v_ad

s=sigmoid(V_update*X_bar);

sigma = [1 ; s(:,1) ];
v_ad = W_update*sigma;

%% Compute v_ad_comp
Z = [ V,zeros(size(V,1),size(W,2));
    zeros(size(W,1),size(V,2)),W];
    
Z_norm = norm(Z,'fro');
Z_max = 2*min(size(W,1),size(W,2) )*min( size(V,1),size(V,2) );
Z_norm_unit = Z_norm;

K_r0= 0.02;
K_r1= 0;
v_r0 = -K_r0*zeta';
v_r1 = -K_r1*(Z_norm+Z_max)*zeta';

v_ad_comp = v_ad + v_r1 +v_r0;


end

== matlab function F16ASYM_Controlled_AoA/P controller + adaptive Crossed NN + AWU+Lim+scheduling   in AoA/Sigmoid /MATLAB Function ==
  data: u input; y output; a input
function y = sigmoid_a(u,a)

y = 2.0 ./ (1.0 + exp(-a*u(1:3)))-1;

== matlab function F16ASYM_Controlled_AoA/Control allocator1/Control allocator: RECONFIG/MATLAB Function ==
  data: Deflections input; Saturations output; Sup_lim input; Inf_lim input
function Saturations = Saturations(Deflections,Sup_lim,Inf_lim)
Saturations=zeros(7,1);

for i=1:7
    
    if Deflections(i)>=Sup_lim(i)
        Saturations(i)=1;
    elseif Deflections(i)<=Inf_lim(i)
        Saturations(i)=-1;
    else
        Saturations(i)=0;
    end
end

== system F16ASYM_Controlled_AoA/Anti-windup Calculation/Anti-windup: Reconfigurable/Moments ==
  C_L : Inport
  C_M : Inport  Port=2
  C_N : Inport  Port=3
  q : Inport  Port=4
  B span : Constant  Value=9.144
  CMA : Constant  Value=3.45
  Divide : Product  Inputs=**
  Divide1 : Product  Inputs=***
  Divide2 : Product  Inputs=**
  Divide3 : Product  Inputs=***
  Divide4 : Product  Inputs=**
  S_w : Constant  Value=27.87
  S_w1 : Constant  Value=27.87
  q1 : InportShadow  Port=4
  L : Outport
  M : Outport  Port=2
  N : Outport  Port=3
  wires:
  Divide4/1 -> M/1  "M"
  Divide3/1 -> Divide4/2
  C_M/1 -> Divide4/1
  CMA/1 -> Divide3/3
  S_w1/1 -> Divide3/2
  q1/1 -> Divide3/1
  Divide2/1 -> N/1  "N"
  C_N/1 -> Divide2/2
  Divide/1 -> L/1  "L"
  Divide1/1 -> Divide/2, Divide2/1
  C_L/1 -> Divide/1
  B span/1 -> Divide1/3
  S_w/1 -> Divide1/2
  q/1 -> Divide1/1

== system F16ASYM_Controlled_AoA/Control allocator/Control allocator: NO RECONF/Leading Edge Flap:Symetric deflection ==
  note: Initialize LF_state with -alpha0 value in degrees!!!!
  note: Same as atmos() in nlplant...c
  note: see NASA Technical Paper 1538, p34
  All_meas : Inport
  Bus Selector : BusSelector  OutputSignals=signal1.Alt meas (m),signal1.V_TAS (m/s),signal1.AoA meas (rad)
  Creating    qbar / ps : Subsystem
  Gain : Gain  Gain=2  SaturateOnIntegerOverflow=on  OutDataTypeStr=Inherit: Same as input  ParamDataTypeStr=Inherit: Same as input
  Gain1 : Gain  Gain=7.25  SaturateOnIntegerOverflow=on  OutDataTypeStr=Inherit: Same as input  ParamDataTypeStr=Inherit: Same as input
  Gain2 : Gain  Gain=1.38  SaturateOnIntegerOverflow=on  OutDataTypeStr=Inherit: Same as input  ParamDataTypeStr=Inherit: Same as input
  LF_state : Integrator  InitialCondition=-trim_state(8)*180/pi
  Sum : Sum  Inputs=-|+|+  SaturateOnIntegerOverflow=on  InputSameDT=on  OutDataTypeStr=Inherit: Same as first input
  Sum1 : Sum  Inputs=|+-  SaturateOnIntegerOverflow=on  InputSameDT=on  OutDataTypeStr=Inherit: Same as first input
  Sum2 : Sum  Inputs=++|  SaturateOnIntegerOverflow=on  InputSameDT=on  OutDataTypeStr=Inherit: Same as first input
  coeff1 : Constant  Value=1.45
  r2d1 : Gain  Gain=180/pi  SaturateOnIntegerOverflow=on  OutDataTypeStr=Inherit: Same as input  ParamDataTypeStr=Inherit: Same as input
  r2d6 : Gain  Gain=9.05  SaturateOnIntegerOverflow=on  OutDataTypeStr=Inherit: Same as input  ParamDataTypeStr=Inherit: Same as input
  delta_lef (deg) : Outport
  wires:
  Bus Selector/3 -> r2d1/1  "<AoA meas (rad)>"
  Bus Selector/1 -> Creating    qbar / ps/1(alt)  "<Alt meas (m)>"
  r2d6/1 -> Sum/1
  Creating    qbar / ps/1(qbar / ps) -> r2d6/1
  Bus Selector/2 -> Creating    qbar / ps/2(V)  "<V_TAS (m/s)>"
  r2d1/1 -> Gain/1, Sum1/1  "alpha deg"
  LF_state/1 -> Sum2/2
  Sum2/1 -> Gain2/1, Sum1/2
  coeff1/1 -> Sum/3
  Gain2/1 -> Sum/2
  Gain/1 -> Sum2/1
  Gain1/1 -> LF_state/1
  Sum1/1 -> Gain1/1
  All_meas/1 -> Bus Selector/1
  Sum/1 -> delta_lef (deg)/1

== system F16ASYM_Controlled_AoA/Control allocator/Control allocator: RECONFIG/Blockades logic: Limits injetor ==
  note: No dynamics for throttle since the engine dynamics is inside the model
  Abs pos limits : Inport
  Last deflection (abs) : Inport  Port=2
  Blockades : Inport  Port=3
  Blockade now : Inport  Port=4
  Block AT INFERIOR LIMIT : Subsystem
  Block AT SUPERIOR LIMIT : Subsystem
  Block NOW INFERIOR LIMIT : Subsystem
  Block NOW SUPERIOR LIMIT : Subsystem
  Inf : Selector  NumberOfDimensions=2  InputPortWidth=3  IndexOptions=Index vector (dialog),Index vector (dialog)  Indices=[1:7],1  OutputSizes=1,1
  Matrix Concatenate : Concatenate  Mode=Multidimensional array  ConcatenateDimension=2
  Sup : Selector  NumberOfDimensions=2  InputPortWidth=3  IndexOptions=Index vector (dialog),Index vector (dialog)  Indices=[1:7],2  OutputSizes=1,1
  Pos limits(abs) : Outport
  wires:
  Last deflection (abs)/1 -> Block NOW SUPERIOR LIMIT/3(Last deflection (abs)), Block NOW INFERIOR LIMIT/3(Last deflection (abs))
  Matrix Concatenate/1 -> Pos limits(abs)/1
  Blockade now/1 -> Block NOW INFERIOR LIMIT/2(Blockade now), Block NOW SUPERIOR LIMIT/2(Blockade now)
  Abs pos limits/1 -> Sup/1, Inf/1
  Blockades/1 -> Block AT INFERIOR LIMIT/2(Blockades), Block AT SUPERIOR LIMIT/2(Blockades)
  Inf/1 -> Block AT INFERIOR LIMIT/1(Limit)
  Sup/1 -> Block AT SUPERIOR LIMIT/1(Limit)
  Block AT INFERIOR LIMIT/1(Reconfig limits) -> Block NOW INFERIOR LIMIT/1(Limit)
  Block AT SUPERIOR LIMIT/1(Reconfig limits) -> Block NOW SUPERIOR LIMIT/1(Limit)
  Block NOW INFERIOR LIMIT/1(Reconfig limits) -> Matrix Concatenate/1
  Block NOW SUPERIOR LIMIT/1(Reconfig limits) -> Matrix Concatenate/2

== system F16ASYM_Controlled_AoA/Control allocator/Control allocator: RECONFIG/Leading Edge Flap:Symetric deflection ==
  note: see NASA Technical Paper 1538, p34
  note: Same as atmos() in nlplant...c
  note: Initialize LF_state with -alpha0 value in degrees!!!!
  All_meas : Inport
  Bus Selector : BusSelector  OutputSignals=signal1.Alt meas (m),signal1.V_TAS (m/s),signal1.AoA meas (rad)
  Creating    qbar / ps : Subsystem
  Gain : Gain  Gain=2  SaturateOnIntegerOverflow=on  OutDataTypeStr=Inherit: Same as input  ParamDataTypeStr=Inherit: Same as input
  Gain1 : Gain  Gain=7.25  SaturateOnIntegerOverflow=on  OutDataTypeStr=Inherit: Same as input  ParamDataTypeStr=Inherit: Same as input
  Gain2 : Gain  Gain=1.38  SaturateOnIntegerOverflow=on  OutDataTypeStr=Inherit: Same as input  ParamDataTypeStr=Inherit: Same as input
  LF_state : Integrator  InitialCondition=-trim_state(8)*180/pi
  Sum : Sum  Inputs=-|+|+  SaturateOnIntegerOverflow=on  InputSameDT=on  OutDataTypeStr=Inherit: Same as first input
  Sum1 : Sum  Inputs=|+-  SaturateOnIntegerOverflow=on  InputSameDT=on  OutDataTypeStr=Inherit: Same as first input
  Sum2 : Sum  Inputs=++|  SaturateOnIntegerOverflow=on  InputSameDT=on  OutDataTypeStr=Inherit: Same as first input
  coeff1 : Constant  Value=1.45
  r2d1 : Gain  Gain=180/pi  SaturateOnIntegerOverflow=on  OutDataTypeStr=Inherit: Same as input  ParamDataTypeStr=Inherit: Same as input
  r2d6 : Gain  Gain=9.05  SaturateOnIntegerOverflow=on  OutDataTypeStr=Inherit: Same as input  ParamDataTypeStr=Inherit: Same as input
  delta_lef (deg) : Outport
  wires:
  Sum/1 -> delta_lef (deg)/1
  All_meas/1 -> Bus Selector/1
  Sum1/1 -> Gain1/1
  Gain1/1 -> LF_state/1
  Gain/1 -> Sum2/1
  Gain2/1 -> Sum/2
  coeff1/1 -> Sum/3
  Sum2/1 -> Sum1/2, Gain2/1
  LF_state/1 -> Sum2/2
  r2d1/1 -> Sum1/1, Gain/1  "alpha deg"
  Bus Selector/2 -> Creating    qbar / ps/2(V)  "<V_TAS (m/s)>"
  Creating    qbar / ps/1(qbar / ps) -> r2d6/1
  r2d6/1 -> Sum/1
  Bus Selector/1 -> Creating    qbar / ps/1(alt)  "<Alt meas (m)>"
  Bus Selector/3 -> r2d1/1  "<AoA meas (rad)>"

== system F16ASYM_Controlled_AoA/Control allocator1/Control allocator: NO RECONF/Leading Edge Flap:Symetric deflection ==
  note: Initialize LF_state with -alpha0 value in degrees!!!!
  note: Same as atmos() in nlplant...c
  note: see NASA Technical Paper 1538, p34
  All_meas : Inport
  Bus Selector : BusSelector  OutputSignals=signal1.Alt meas (m),signal1.V_TAS (m/s),signal1.AoA meas (rad)
  Creating    qbar / ps : Subsystem
  Gain : Gain  Gain=2  SaturateOnIntegerOverflow=on  OutDataTypeStr=Inherit: Same as input  ParamDataTypeStr=Inherit: Same as input
  Gain1 : Gain  Gain=7.25  SaturateOnIntegerOverflow=on  OutDataTypeStr=Inherit: Same as input  ParamDataTypeStr=Inherit: Same as input
  Gain2 : Gain  Gain=1.38  SaturateOnIntegerOverflow=on  OutDataTypeStr=Inherit: Same as input  ParamDataTypeStr=Inherit: Same as input
  LF_state : Integrator  InitialCondition=-trim_state(8)*180/pi
  Sum : Sum  Inputs=-|+|+  SaturateOnIntegerOverflow=on  InputSameDT=on  OutDataTypeStr=Inherit: Same as first input
  Sum1 : Sum  Inputs=|+-  SaturateOnIntegerOverflow=on  InputSameDT=on  OutDataTypeStr=Inherit: Same as first input
  Sum2 : Sum  Inputs=++|  SaturateOnIntegerOverflow=on  InputSameDT=on  OutDataTypeStr=Inherit: Same as first input
  coeff1 : Constant  Value=1.45
  r2d1 : Gain  Gain=180/pi  SaturateOnIntegerOverflow=on  OutDataTypeStr=Inherit: Same as input  ParamDataTypeStr=Inherit: Same as input
  r2d6 : Gain  Gain=9.05  SaturateOnIntegerOverflow=on  OutDataTypeStr=Inherit: Same as input  ParamDataTypeStr=Inherit: Same as input
  delta_lef (deg) : Outport
  wires:
  Bus Selector/3 -> r2d1/1  "<AoA meas (rad)>"
  Bus Selector/1 -> Creating    qbar / ps/1(alt)  "<Alt meas (m)>"
  r2d6/1 -> Sum/1
  Creating    qbar / ps/1(qbar / ps) -> r2d6/1
  Bus Selector/2 -> Creating    qbar / ps/2(V)  "<V_TAS (m/s)>"
  r2d1/1 -> Gain/1, Sum1/1  "alpha deg"
  LF_state/1 -> Sum2/2
  Sum2/1 -> Gain2/1, Sum1/2
  coeff1/1 -> Sum/3
  Gain2/1 -> Sum/2
  Gain/1 -> Sum2/1
  Gain1/1 -> LF_state/1
  Sum1/1 -> Gain1/1
  All_meas/1 -> Bus Selector/1
  Sum/1 -> delta_lef (deg)/1

== system F16ASYM_Controlled_AoA/Control allocator1/Control allocator: RECONFIG/Blockades logic: Limits injetor ==
  note: 1st order models here to avoid coupling
  note: No dynamics for throttle since the engine dynamics is inside the model
  Abs pos limits : Inport
  Last deflection (abs) : Inport  Port=2
  Blockades : Inport  Port=3
  Blockade now : Inport  Port=4
  1st order model : Subsystem  mask{tau=T_sim*4, y_i=[-24,-24,-21,-21,-29,0,0]}
      mask prompts: tau "1st order time constant (tau)"; y_i "Initial state"
      mask init:
      | K_ref=1/tau;
      mask Display:
      | [y,t]=step(tf([K_ref],[1 K_ref]));
      | pos = get_param(gcb, 'Position');
      | width = pos(3) - pos(1);
      | height = pos(4) - pos(2);
      | t = t.*width/max(t);
      | y=y.*height/max(y);
      | plot(t,y);
      | 
      | 
      | text(0.5*width,0.92*height,['tau=',num2str(tau)]);
      | 
      | dpoly([K_ref],[1 K_ref], 's')
  1st order model1 : Subsystem  mask{tau=T_sim*4, y_i=[24,24,21,21,29,25,25]}
      mask prompts: tau "1st order time constant (tau)"; y_i "Initial state"
      mask init:
      | K_ref=1/tau;
      mask Display:
      | [y,t]=step(tf([K_ref],[1 K_ref]));
      | pos = get_param(gcb, 'Position');
      | width = pos(3) - pos(1);
      | height = pos(4) - pos(2);
      | t = t.*width/max(t);
      | y=y.*height/max(y);
      | plot(t,y);
      | 
      | 
      | text(0.5*width,0.92*height,['tau=',num2str(tau)]);
      | 
      | dpoly([K_ref],[1 K_ref], 's')
  Add : Sum
  Block AT INFERIOR LIMIT : Subsystem
  Block AT SUPERIOR LIMIT : Subsystem
  Block NOW INFERIOR LIMIT : Subsystem
  Block NOW SUPERIOR LIMIT : Subsystem
  Inf : Selector  NumberOfDimensions=2  InputPortWidth=3  IndexOptions=Index vector (dialog),Index vector (dialog)  Indices=[1:7],1  OutputSizes=1,1
  Matrix Concatenate : Concatenate  Mode=Multidimensional array  ConcatenateDimension=2
  Saturation : Saturate  UpperLimit=1  LowerLimit=0
  Sup : Selector  NumberOfDimensions=2  InputPortWidth=3  IndexOptions=Index vector (dialog),Index vector (dialog)  Indices=[1:7],2  OutputSizes=1,1
  Pos limits(abs) : Outport
  Surf blocked : Outport  Port=2
  wires:
  Last deflection (abs)/1 -> Block NOW SUPERIOR LIMIT/3(Last deflection (abs)), Block NOW INFERIOR LIMIT/3(Last deflection (abs))
  Matrix Concatenate/1 -> Pos limits(abs)/1
  Blockade now/1 -> Block NOW SUPERIOR LIMIT/2(Blockade now), Block NOW INFERIOR LIMIT/2(Blockade now), Add/2
  Abs pos limits/1 -> Sup/1, Inf/1
  Blockades/1 -> Block AT INFERIOR LIMIT/2(Blockades), Block AT SUPERIOR LIMIT/2(Blockades)
  Inf/1 -> Block AT INFERIOR LIMIT/1(Limit)
  Sup/1 -> Block AT SUPERIOR LIMIT/1(Limit)
  Block AT INFERIOR LIMIT/1(Reconfig limits) -> Block NOW INFERIOR LIMIT/1(Limit)
  Block AT SUPERIOR LIMIT/1(Reconfig limits) -> Block NOW SUPERIOR LIMIT/1(Limit)
  1st order model/1(y_out) -> Matrix Concatenate/1
  Block NOW SUPERIOR LIMIT/1(Reconfig limits) -> 1st order model1/1(y_in)
  Block AT INFERIOR LIMIT/2(Surf blocked) -> Add/1
  Add/1 -> Saturation/1
  Saturation/1 -> Surf blocked/1
  Block NOW INFERIOR LIMIT/1(Reconfig limits) -> 1st order model/1(y_in)
  1st order model1/1(y_out) -> Matrix Concatenate/2

== system F16ASYM_Controlled_AoA/Control allocator1/Control allocator: RECONFIG/Leading Edge Flap:Symetric deflection ==
  note: see NASA Technical Paper 1538, p34
  note: Same as atmos() in nlplant...c
  note: Initialize LF_state with -alpha0 value in degrees!!!!
  All_meas : Inport
  Bus Selector : BusSelector  OutputSignals=signal1.Alt meas (m),signal1.V_TAS (m/s),signal1.AoA meas (rad)
  Creating    qbar / ps : Subsystem
  Gain : Gain  Gain=2  SaturateOnIntegerOverflow=on  OutDataTypeStr=Inherit: Same as input  ParamDataTypeStr=Inherit: Same as input
  Gain1 : Gain  Gain=7.25  SaturateOnIntegerOverflow=on  OutDataTypeStr=Inherit: Same as input  ParamDataTypeStr=Inherit: Same as input
  Gain2 : Gain  Gain=1.38  SaturateOnIntegerOverflow=on  OutDataTypeStr=Inherit: Same as input  ParamDataTypeStr=Inherit: Same as input
  LF_state : Integrator  InitialCondition=-trim_state(8)*180/pi
  Sum : Sum  Inputs=-|+|+  SaturateOnIntegerOverflow=on  InputSameDT=on  OutDataTypeStr=Inherit: Same as first input
  Sum1 : Sum  Inputs=|+-  SaturateOnIntegerOverflow=on  InputSameDT=on  OutDataTypeStr=Inherit: Same as first input
  Sum2 : Sum  Inputs=++|  SaturateOnIntegerOverflow=on  InputSameDT=on  OutDataTypeStr=Inherit: Same as first input
  coeff1 : Constant  Value=1.45
  r2d1 : Gain  Gain=180/pi  SaturateOnIntegerOverflow=on  OutDataTypeStr=Inherit: Same as input  ParamDataTypeStr=Inherit: Same as input
  r2d6 : Gain  Gain=9.05  SaturateOnIntegerOverflow=on  OutDataTypeStr=Inherit: Same as input  ParamDataTypeStr=Inherit: Same as input
  delta_lef (deg) : Outport
  wires:
  Sum/1 -> delta_lef (deg)/1
  All_meas/1 -> Bus Selector/1
  Sum1/1 -> Gain1/1
  Gain1/1 -> LF_state/1
  Gain/1 -> Sum2/1
  Gain2/1 -> Sum/2
  coeff1/1 -> Sum/3
  Sum2/1 -> Sum1/2, Gain2/1
  LF_state/1 -> Sum2/2
  r2d1/1 -> Sum1/1, Gain/1  "alpha deg"
  Bus Selector/2 -> Creating    qbar / ps/2(V)  "<V_TAS (m/s)>"
  Creating    qbar / ps/1(qbar / ps) -> r2d6/1
  r2d6/1 -> Sum/1
  Bus Selector/1 -> Creating    qbar / ps/1(alt)  "<Alt meas (m)>"
  Bus Selector/3 -> r2d1/1  "<AoA meas (rad)>"
